simulink model "TakeOffAnalysis"  (R2021a)
settings: Solver=ode5  StartTime=0.0  StopTime=10  FixedStep=0.01  RelTol=1e-3
model workspace (MAT data in the model file):
  CD = 0
  CL = 0
  mass = 3.5
libraries: simulink_extras x1
settings Model: Creator=PC  LastModifiedBy=PC

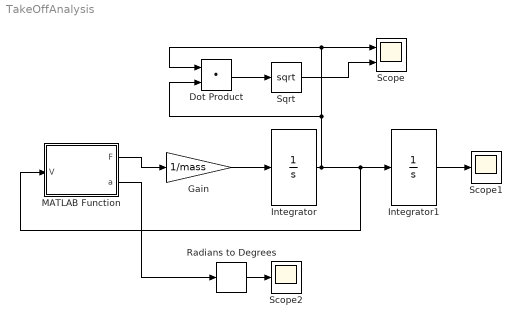
== system TakeOffAnalysis ==
  Dot Product : DotProduct  InputSameDT=on  OutDataTypeStr=Inherit: Inherit via internal rule
  Gain : Gain  Gain=1/mass
  Integrator : Integrator  InitialCondition=[7;0]
  Integrator1 : Integrator  InitialCondition=[0;-2]
  MATLAB Function : MATLAB Function  TreatAsAtomicUnit=on
  Radians to Degrees : simulink_extras/Transformations/Radians to Degrees
  Scope : Scope  NumInputPorts=2
  Scope1 : Scope
  Scope2 : Scope
  Sqrt : Sqrt  SaturateOnIntegerOverflow=on
  wires:
  MATLAB Function/1(F) -> Gain/1
  Gain/1 -> Integrator/1
  Integrator/1 -> Integrator1/1, MATLAB Function/1(V), Dot Product/1, Scope/1, Dot Product/2
  Integrator1/1 -> Scope1/1
  MATLAB Function/2(a) -> Radians to Degrees/1
  Radians to Degrees/1 -> Scope2/1
  Dot Product/1 -> Sqrt/1
  Sqrt/1 -> Scope/2

== matlab function TakeOffAnalysis/MATLAB Function ==
  data: V input; F output; a output
function [F, a] = fcn(V)
S = 0.340;
M = 3.5;
T = 20;
rho = 1.225;
g = 9.81;
CD = 0.045;
CL = 0.47;
CLa = 5;
C = [CD; CL];

a = atan(V(2)/V(1));

D = rho*(dot(V, V))/2 * S * CD;
L = rho*(dot(V, V))/2 * S * (CL+CLa*a);

F = [T - D*cos(a) - L*sin(a);
     M*g + D*sin(a) - L*cos(a)];
